simulink model "LTDung_Library2222222"  (R2016a)
settings: Solver=VariableStepAuto  SolverMode=SingleTasking  StartTime=0.0  StopTime=10.0  RelTol=1e-3
undefined symbols (not defined in the file): a, b, c, d, DiscIntNeverNeededParam, f, g, p, pe, Ts
libraries: simulink x4, powerlib_extras x2, powerlib x1
settings Model: Creator=Admin  LastModifiedBy=? ? ?
settings DebuggingCC: SFUnexpectedBacktrackingDiag=error  SFNoUnconditionalDefaultTransitionDiag=error
settings GRTTargetCC: TargetLangStandard=C99 (ISO)  GeneratePreprocessorConditionals=Use local settings
settings ConfigComp: CovMetricSettings=dwe  CovHtmlReporting=off  CovSaveCumulativeToWorkspaceVar=off  CovSaveSingleToWorkspaceVar=off  CovExternalEMLEnable=on

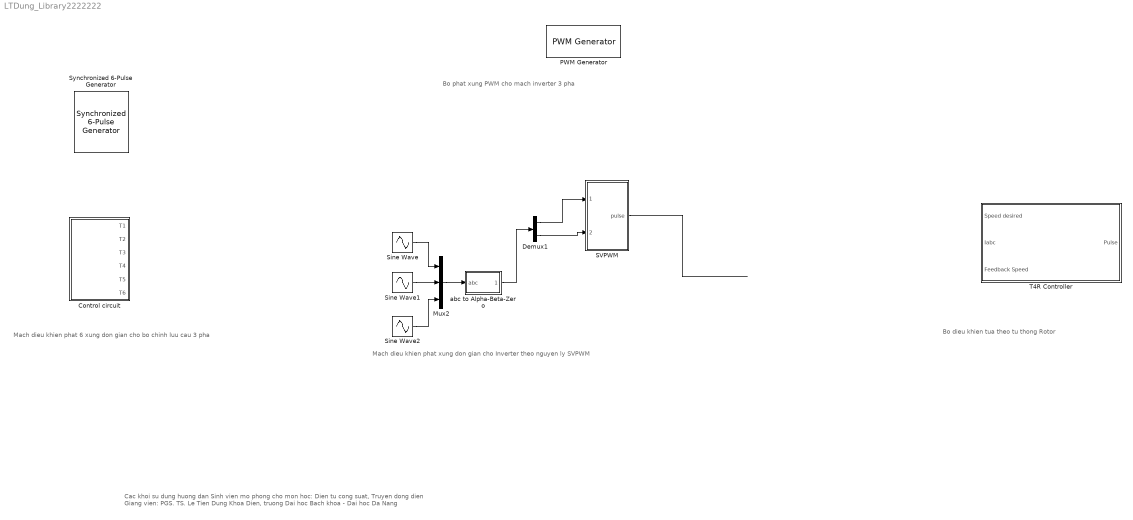
== system LTDung_Library2222222 ==
  note: Cac khoi su dung huong dan Sinh vien mo phong cho mon hoc: Dien tu cong suat, Truyen dong dien
      |
      | Giang vien: PGS. TS. Le Tien Dung
      | Khoa Dien, truong Dai hoc Bach khoa - Dai hoc Da Nang
  note: Mach dieu khien phat xung don gian cho Inverter theo nguyen ly SVPWM
  note: Mach dieu khien phat 6 xung don gian
      | cho bo chinh luu cau 3 pha
  note: Bo dieu khien tua theo tu thong Rotor
  note: Bo phat xung PWM cho mach inverter 3 pha
  Control circuit : Subsystem
  Demux1 : Demux  Outputs=2
  Mux2 : Mux  Inputs=3
  PWM Generator : powerlib_extras/Control  Blocks/PWM Generator  GeneratorMode="3-arm  bridge (6 pulses)"  Fc=5000  Internal=on  mIndex=1  Freq=50  Phase=0
  SVPWM : Subsystem
  Sine Wave : Sin  Amplitude=220*sqrt(2)  Frequency=50  SampleTime=0
  Sine Wave1 : Sin  Amplitude=220*sqrt(2)  Frequency=50  Phase=-2*pi/3  SampleTime=0
  Sine Wave2 : Sin  Amplitude=220*sqrt(2)  Frequency=50  Phase=-4*pi/3  SampleTime=0
  Synchronized 6-Pulse Generator : powerlib_extras/Control  Blocks/Synchronized 6-Pulse Generator  freq=50  pwidth=10  Double_Pulse=off
  T4R Controller : Subsystem
  abc to Alpha-Beta-Zero : Subsystem  AncestorBlock=powerlib_meascontrol/Transformations/abc to Alpha-Beta-Zero  DialogController=POWERSYS.PowerSysDialog  mask(abc to Alpha-Beta-Zero Transformation){}
      mask help: Perform a Clarke transformation from a three-phase (abc) signal to a alpha-beta-zero stationary reference frame.
      mask Help: helpview(psbhelp);
      mask Display:
      | plot([0 1], [0,1])
      | text(0.15,0.7,'abc')
      | text(0.55, 0.3,'\alpha\beta0','texmode','on')
  wires:
  Sine Wave/1 -> Mux2/1
  Demux1/1 -> SVPWM/1(Ualpha)
  abc to Alpha-Beta-Zero/1(al_be) -> Demux1/1
  Sine Wave1/1 -> Mux2/2
  Sine Wave2/1 -> Mux2/3
  Demux1/2 -> SVPWM/2(Ubeta)
  Mux2/1 -> abc to Alpha-Beta-Zero/1(abc)
  SVPWM/1(pulse) -> ?

== system LTDung_Library2222222/Control circuit ==
  Discription : Subsystem
  P1 : DiscretePulseGenerator  PulseType=Time based  Period=1/f  PulseWidth=p  PhaseDelay=((pe*a)/360)
  P2 : DiscretePulseGenerator  PulseType=Time based  Period=1/f  PulseWidth=p  PhaseDelay=((pe*b)/360)
  P3 : DiscretePulseGenerator  PulseType=Time based  Period=1/f  PulseWidth=p  PhaseDelay=((pe*c)/360)
  P4 : DiscretePulseGenerator  PulseType=Time based  Period=1/f  PulseWidth=p  PhaseDelay=((pe*d)/360)
  P5 : DiscretePulseGenerator  PulseType=Time based  Period=1/f  PulseWidth=p  PhaseDelay=((pe*e)/360)
  P6 : DiscretePulseGenerator  PulseType=Time based  Period=1/f  PulseWidth=p  PhaseDelay=((pe*g)/360)
  T1 : Outport
  T2 : Outport  Port=2
  T3 : Outport  Port=3
  T4 : Outport  Port=4
  T5 : Outport  Port=5
  T6 : Outport  Port=6
  wires:
  P4/1 -> T4/1
  P2/1 -> T2/1
  P6/1 -> T6/1
  P1/1 -> T1/1
  P5/1 -> T5/1
  P3/1 -> T3/1

== system LTDung_Library2222222/SVPWM ==
  Ualpha : Inport
  Ubeta : Inport  Port=2
  N1 : Subsystem
  Scope : Scope
  Scope1 : Scope
  Scope3 : Scope  NumInputPorts=2
  Scope6 : Scope
  Subsystem : Subsystem
  Subsystem1 : Subsystem
  T : Constant  Value=0.0001
  Udc : Constant  Value=620
  X.Y.Z : Subsystem
  produce PWM : Subsystem
  pulse : Outport
  wires:
  T/1 -> X.Y.Z/1(T), Subsystem1/3(T), Subsystem/5(T)
  Udc/1 -> X.Y.Z/4(Udc)
  N1/1(N) -> Subsystem/1(N), Subsystem1/4(N), Scope1/1
  X.Y.Z/1(X) -> Subsystem/2(X)
  X.Y.Z/2(Y) -> Subsystem/3(Y)
  X.Y.Z/3(Z) -> Subsystem/4(Z)
  Subsystem1/1(Tcm1) -> produce PWM/1(Tcm1), Scope/1
  Subsystem1/2(Tcm2) -> produce PWM/2(Tcm2)
  Subsystem1/3(Tcm3) -> produce PWM/3(Tcm3)
  Ualpha/1 -> Scope3/1, X.Y.Z/2(Ualfa), N1/1(Ualpha)
  Subsystem/1(T1) -> Subsystem1/1(T1), Scope6/1
  Subsystem/2(T2) -> Subsystem1/2(T2)
  Ubeta/1 -> X.Y.Z/3(Ubeta), N1/2(Ubeta), Scope3/2
  produce PWM/1(pulse) -> pulse/1

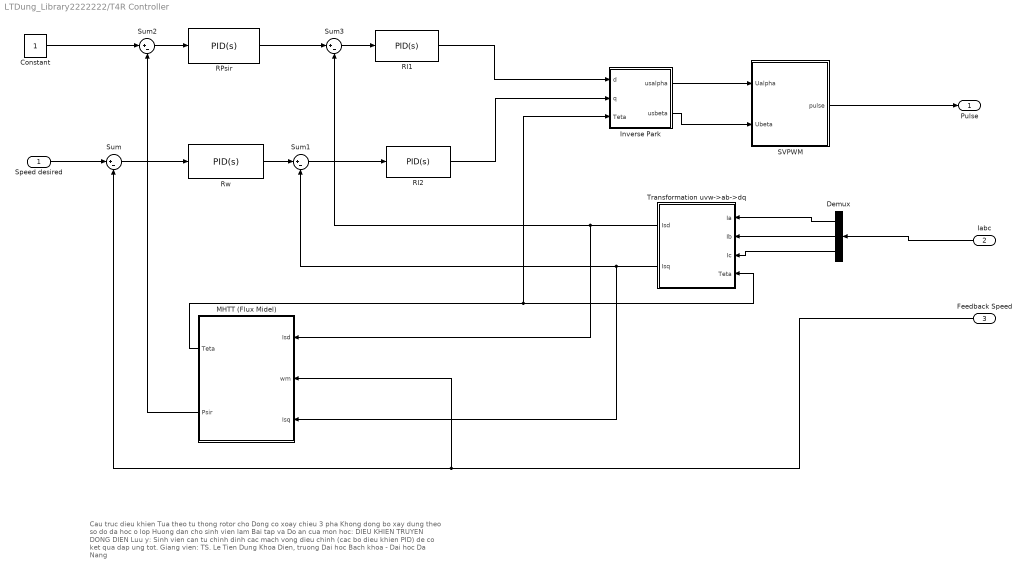
== system LTDung_Library2222222/T4R Controller ==
  note: Cau truc dieu khien Tua theo tu thong rotor cho Dong co xoay chieu 3 pha Khong dong bo xay dung theo so do da hoc o lop
      | Huong dan cho sinh vien lam Bai tap va Do an cua mon hoc: DIEU KHIEN TRUYEN DONG DIEN
      |
      | Luu y: Sinh vien can tu chinh dinh cac mach vong dieu chinh (cac bo dieu khien PID) de co ket qua dap ung tot.
      |
      | Giang vien: TS. Le Tien Dung
      | Khoa Dien, truong Dai hoc Bach khoa - Dai hoc Da Nang
  Speed desired : Inport
  Iabc : Inport  Port=2
  Feedback Speed : Inport  Port=3
  Constant : Constant
  Demux : Demux  Outputs=3
  Inverse Park : Subsystem
  MHTT (Flux Midel) : Subsystem
  RI1 : simulink/Continuous/PID Controller  Controller=PID  Form=Parallel  TimeDomain=Continuous-time  SampleTime=-1  IntegratorMethod=Forward Euler  FilterMethod=Forward Euler  ControllerParametersSource=internal  P=1  I=1  D=0  UseFilter=on  N=100  InitialConditionSource=internal  InitialConditionForIntegrator=0  InitialConditionForFilter=0  DifferentiatorICPrevScaledInput=0  ExternalReset=none  TrackingMode=off  Kt=1  LimitOutput=off  UpperSaturationLimit=inf  LowerSaturationLimit=-inf  LinearizeAsGain=on  AntiWindupMode=none  Kb=1  POutMin=[]  POutMax=[]  IOutMin=[]  IOutMax=[]  DOutMin=[]  DOutMax=[]  NOutMin=[]  NOutMax=[]  SumOutMin=[]  SumOutMax=[]  SaturationOutMin=[]  SaturationOutMax=[]  PParamMin=[]  PParamMax=[]  IParamMin=[]  IParamMax=[]  DParamMin=[]  DParamMax=[]  NParamMin=[]  NParamMax=[]  KbParamMin=[]  KbParamMax=[]  KtParamMin=[]  KtParamMax=[]  KbOutMin=[]  KbOutMax=[]  KtOutMin=[]  KtOutMax=[]  IntegratorOutMin=[]  IntegratorOutMax=[]  FilterOutMin=[]  FilterOutMax=[]  SumI1OutMin=[]  SumI1OutMax=[]  SumI2OutMin=[]  SumI2OutMax=[]  SumI3OutMin=[]  SumI3OutMax=[]  SumDOutMin=[]  SumDOutMax=[]  DifferentiatorOutMin=[]  DifferentiatorOutMax=[]  IntegratorContinuousStateAttributes=''  IntegratorStateMustResolveToSignalObject=off  IntegratorRTWStateStorageClass=Auto  FilterContinuousStateAttributes=''  FilterStateMustResolveToSignalObject=off  FilterRTWStateStorageClass=Auto
  RI2 : simulink/Continuous/PID Controller  Controller=PID  Form=Parallel  TimeDomain=Continuous-time  SampleTime=-1  IntegratorMethod=Forward Euler  FilterMethod=Forward Euler  ControllerParametersSource=internal  P=1  I=1  D=0  UseFilter=on  N=100  InitialConditionSource=internal  InitialConditionForIntegrator=0  InitialConditionForFilter=0  DifferentiatorICPrevScaledInput=0  ExternalReset=none  TrackingMode=off  Kt=1  LimitOutput=off  UpperSaturationLimit=inf  LowerSaturationLimit=-inf  LinearizeAsGain=on  AntiWindupMode=none  Kb=1  POutMin=[]  POutMax=[]  IOutMin=[]  IOutMax=[]  DOutMin=[]  DOutMax=[]  NOutMin=[]  NOutMax=[]  SumOutMin=[]  SumOutMax=[]  SaturationOutMin=[]  SaturationOutMax=[]  PParamMin=[]  PParamMax=[]  IParamMin=[]  IParamMax=[]  DParamMin=[]  DParamMax=[]  NParamMin=[]  NParamMax=[]  KbParamMin=[]  KbParamMax=[]  KtParamMin=[]  KtParamMax=[]  KbOutMin=[]  KbOutMax=[]  KtOutMin=[]  KtOutMax=[]  IntegratorOutMin=[]  IntegratorOutMax=[]  FilterOutMin=[]  FilterOutMax=[]  SumI1OutMin=[]  SumI1OutMax=[]  SumI2OutMin=[]  SumI2OutMax=[]  SumI3OutMin=[]  SumI3OutMax=[]  SumDOutMin=[]  SumDOutMax=[]  DifferentiatorOutMin=[]  DifferentiatorOutMax=[]  IntegratorContinuousStateAttributes=''  IntegratorStateMustResolveToSignalObject=off  IntegratorRTWStateStorageClass=Auto  FilterContinuousStateAttributes=''  FilterStateMustResolveToSignalObject=off  FilterRTWStateStorageClass=Auto
  RPsir : simulink/Continuous/PID Controller  Controller=PID  Form=Parallel  TimeDomain=Continuous-time  SampleTime=-1  IntegratorMethod=Forward Euler  FilterMethod=Forward Euler  ControllerParametersSource=internal  P=1  I=1  D=0  UseFilter=on  N=100  InitialConditionSource=internal  InitialConditionForIntegrator=0  InitialConditionForFilter=0  DifferentiatorICPrevScaledInput=0  ExternalReset=none  TrackingMode=off  Kt=1  LimitOutput=off  UpperSaturationLimit=inf  LowerSaturationLimit=-inf  LinearizeAsGain=on  AntiWindupMode=none  Kb=1  POutMin=[]  POutMax=[]  IOutMin=[]  IOutMax=[]  DOutMin=[]  DOutMax=[]  NOutMin=[]  NOutMax=[]  SumOutMin=[]  SumOutMax=[]  SaturationOutMin=[]  SaturationOutMax=[]  PParamMin=[]  PParamMax=[]  IParamMin=[]  IParamMax=[]  DParamMin=[]  DParamMax=[]  NParamMin=[]  NParamMax=[]  KbParamMin=[]  KbParamMax=[]  KtParamMin=[]  KtParamMax=[]  KbOutMin=[]  KbOutMax=[]  KtOutMin=[]  KtOutMax=[]  IntegratorOutMin=[]  IntegratorOutMax=[]  FilterOutMin=[]  FilterOutMax=[]  SumI1OutMin=[]  SumI1OutMax=[]  SumI2OutMin=[]  SumI2OutMax=[]  SumI3OutMin=[]  SumI3OutMax=[]  SumDOutMin=[]  SumDOutMax=[]  DifferentiatorOutMin=[]  DifferentiatorOutMax=[]  IntegratorContinuousStateAttributes=''  IntegratorStateMustResolveToSignalObject=off  IntegratorRTWStateStorageClass=Auto  FilterContinuousStateAttributes=''  FilterStateMustResolveToSignalObject=off  FilterRTWStateStorageClass=Auto
  Rw : simulink/Continuous/PID Controller  Controller=PID  Form=Parallel  TimeDomain=Continuous-time  SampleTime=-1  IntegratorMethod=Forward Euler  FilterMethod=Forward Euler  ControllerParametersSource=internal  P=1  I=1  D=0  UseFilter=on  N=100  InitialConditionSource=internal  InitialConditionForIntegrator=0  InitialConditionForFilter=0  DifferentiatorICPrevScaledInput=0  ExternalReset=none  TrackingMode=off  Kt=1  LimitOutput=off  UpperSaturationLimit=inf  LowerSaturationLimit=-inf  LinearizeAsGain=on  AntiWindupMode=none  Kb=1  POutMin=[]  POutMax=[]  IOutMin=[]  IOutMax=[]  DOutMin=[]  DOutMax=[]  NOutMin=[]  NOutMax=[]  SumOutMin=[]  SumOutMax=[]  SaturationOutMin=[]  SaturationOutMax=[]  PParamMin=[]  PParamMax=[]  IParamMin=[]  IParamMax=[]  DParamMin=[]  DParamMax=[]  NParamMin=[]  NParamMax=[]  KbParamMin=[]  KbParamMax=[]  KtParamMin=[]  KtParamMax=[]  KbOutMin=[]  KbOutMax=[]  KtOutMin=[]  KtOutMax=[]  IntegratorOutMin=[]  IntegratorOutMax=[]  FilterOutMin=[]  FilterOutMax=[]  SumI1OutMin=[]  SumI1OutMax=[]  SumI2OutMin=[]  SumI2OutMax=[]  SumI3OutMin=[]  SumI3OutMax=[]  SumDOutMin=[]  SumDOutMax=[]  DifferentiatorOutMin=[]  DifferentiatorOutMax=[]  IntegratorContinuousStateAttributes=''  IntegratorStateMustResolveToSignalObject=off  IntegratorRTWStateStorageClass=Auto  FilterContinuousStateAttributes=''  FilterStateMustResolveToSignalObject=off  FilterRTWStateStorageClass=Auto
  SVPWM : Subsystem
  Sum{,1..3} (4 alike) : Sum  Inputs=|+-
  Transformation uvw->ab->dq : Subsystem
  Pulse : Outport
  wires:
  Speed desired/1 -> Sum/1
  Sum/1 -> Rw/1
  Rw/1 -> Sum1/1
  Sum1/1 -> RI2/1
  RI2/1 -> Inverse Park/2(q)
  Constant/1 -> Sum2/1
  Sum2/1 -> RPsir/1
  RPsir/1 -> Sum3/1
  Sum3/1 -> RI1/1
  RI1/1 -> Inverse Park/1(d)
  Inverse Park/1(usalpha) -> SVPWM/1(Ualpha)
  Inverse Park/2(usbeta) -> SVPWM/2(Ubeta)
  SVPWM/1(pulse) -> Pulse/1
  Feedback Speed/1 -> MHTT (Flux Midel)/2(wm), Sum/2
  Demux/1 -> Transformation uvw->ab->dq/1(Ia)
  Demux/2 -> Transformation uvw->ab->dq/2(Ib)
  Iabc/1 -> Demux/1
  Demux/3 -> Transformation uvw->ab->dq/3(Ic)
  MHTT (Flux Midel)/2(Psir) -> Sum2/2
  MHTT (Flux Midel)/1(Teta) -> Transformation uvw->ab->dq/4(Teta), Inverse Park/3(Teta)
  Transformation uvw->ab->dq/2(Isq) -> MHTT (Flux Midel)/3(Isq), Sum1/2
  Transformation uvw->ab->dq/1(Isd) -> MHTT (Flux Midel)/1(Isd), Sum3/2

== system LTDung_Library2222222/abc to Alpha-Beta-Zero ==
  abc : Inport  PortDimensions=3
  Gain3 : Gain  Gain="[ 1   -1/2   -1/2; 0   sqrt(3)/2   -sqrt(3)/2]"  Multiplication=Matrix(K*u) (u vector)  SaturateOnIntegerOverflow=on  OutDataTypeStr=Inherit: Same as input  ParamDataTypeStr=Inherit: Same as input
  al_be : Outport
  wires:
  abc/1 -> Gain3/1
  Gain3/1 -> al_be/1

== system LTDung_Library2222222/Control circuit/Discription ==
  note: Equation
      |
      | period	= 1/fundamental frequency
      | 		= 1/50
      |
      | phase delay= (period*degree)/360
      |
      | eg	= ((0.02*60)/360)
  note: a=0
      | b=60
      | c=120
      | d=180
      | e=240
      | g=300
  powergui : powerlib/powergui  Priority=1  SimulationMode=Continuous  SampleTime=50e-6  frequency=60  Iterations=50  frequencyindice=0  Pbase=100e6  ErrMax=1e-4  UnitsV=kV  UnitsW=MW  buscounter=0  FunctionMessages=off  echomessages=off  EnableUseOfTLC=off  CurrentSourceSwitches=off  DisableSnubberDevices=off  DisableRonSwitches=off  DisableVfSwitches=off  DisplayEquations=off  SolverType=Tustin/Backward Euler (TBE)  Interpol=off  ExternalGateDelay=off  methode=off  Ts=100  x0status=blocks  SPID=on  SwTol=0  HookPort=off  RestoreLinks=warning  ResistiveCurrentMeasurement=off  Frange=[0:2:500]  Ylog=off  Xlog=on  ShowGrid=off  save=off  variable=ZData  structure=GG  ZoomFFT=off  StartTime=0.02  cycles=1  DisplayStyle=1  fundamental=25  FreqAxis=on  MaxFrequency=1000  frequencyindicesteady=1  RmsSteady=1  display=off

== system LTDung_Library2222222/SVPWM/N1 ==
  Ualpha : Inport
  Ubeta : Inport  Port=2
  Constant : Constant
  Constant1 : Constant  Value=0
  Gain : Gain  Gain=1.732
  Gain1 : Gain  Gain=-1.732
  Gain2 : Gain  Gain=2
  Gain3 : Gain  Gain=4
  Sum : Sum  Inputs=|-+
  Sum1 : Sum  Inputs=|-+
  Sum2 : Sum  Inputs=|+++
  Switch : Switch
  Switch1 : Switch
  Switch2 : Switch
  N : Outport
  wires:
  Ubeta/1 -> Switch/2, Sum/1, Sum1/1
  Constant/1 -> Switch/1, Switch2/1, Switch1/1
  Ualpha/1 -> Gain1/1, Gain/1
  Gain/1 -> Sum/2
  Sum/1 -> Switch1/2
  Sum1/1 -> Switch2/2
  Gain1/1 -> Sum1/2
  Constant1/1 -> Switch/3, Switch1/3, Switch2/3
  Switch1/1 -> Gain2/1
  Switch2/1 -> Gain3/1
  Gain2/1 -> Sum2/2
  Switch/1 -> Sum2/1
  Gain3/1 -> Sum2/3
  Sum2/1 -> N/1

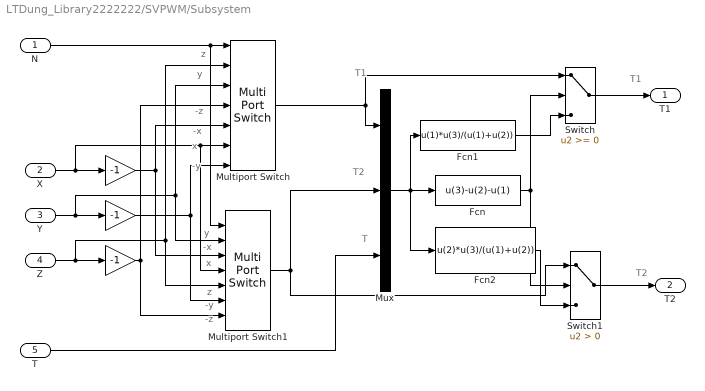
== system LTDung_Library2222222/SVPWM/Subsystem ==
  note: z
  note: y
  note: -z
  note: -x
  note: x
  note: -y
  note: y
  note: -x
  note: x
  note: z
  note: -y
  note: -z
  note: T1
  note: T2
  note: T
  note: T1
  note: T2
  N : Inport
  X : Inport  Port=2
  Y : Inport  Port=3
  Z : Inport  Port=4
  T : Inport  Port=5
  " " : Gain  Gain=-1
  "  " : Gain  Gain=-1
  "    " : Gain  Gain=-1
  Fcn : Fcn  Expr=u(3)-u(2)-u(1)
  Fcn1 : Fcn  Expr=u(1)*u(3)/(u(1)+u(2))
  Fcn2 : Fcn  Expr=u(2)*u(3)/(u(1)+u(2))
  Multiport Switch : MultiPortSwitch  Inputs=6
  Multiport Switch1 : MultiPortSwitch  Inputs=6
  Mux : Mux  Inputs=3
  Switch : Switch
  Switch1 : Switch  Criteria=u2 > Threshold
  T1 : Outport
  T2 : Outport  Port=2
  wires:
  N/1 -> Multiport Switch1/1, Multiport Switch/1
  X/1 -> Multiport Switch1/4, Multiport Switch/6, " "/1
  Y/1 -> Multiport Switch1/2, Multiport Switch/3, "  "/1
  Z/1 -> Multiport Switch1/5, Multiport Switch/2, "    "/1
  "    "/1 -> Multiport Switch1/7, Multiport Switch/4
  "  "/1 -> Multiport Switch/7, Multiport Switch1/6
  " "/1 -> Multiport Switch/5, Multiport Switch1/3
  Multiport Switch/1 -> Mux/1, Switch/1
  Multiport Switch1/1 -> Switch1/1, Mux/2
  T/1 -> Mux/3
  Mux/1 -> Fcn/1, Fcn1/1, Fcn2/1
  Fcn/1 -> Switch/2, Switch1/2
  Fcn1/1 -> Switch/3
  Fcn2/1 -> Switch1/3
  Switch/1 -> T1/1
  Switch1/1 -> T2/1

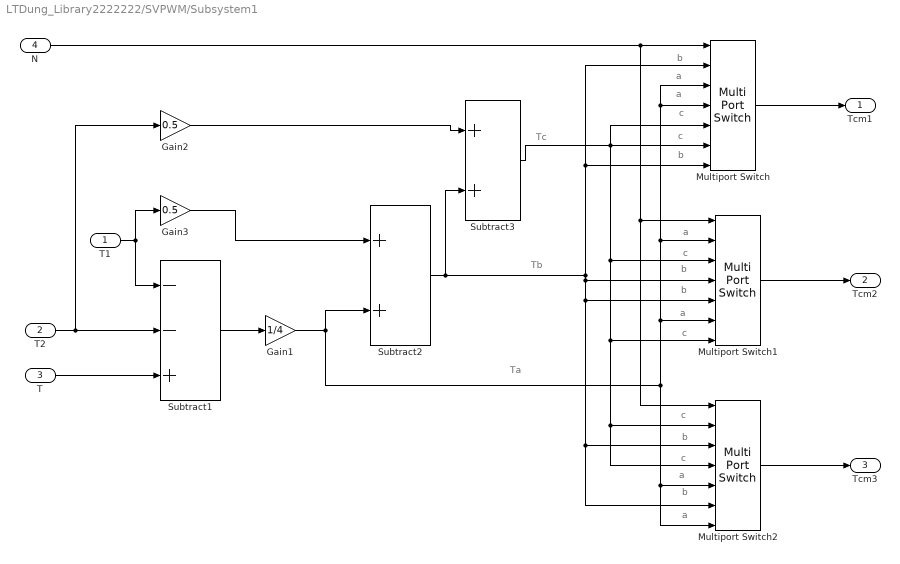
== system LTDung_Library2222222/SVPWM/Subsystem1 ==
  note: Ta
  note: Tb
  note: Tc
  note: b
  note: a
  note: a
  note: c
  note: c
  note: b
  note: a
  note: c
  note: b
  note: b
  note: a
  note: c
  note: c
  note: b
  note: c
  note: a
  note: b
  note: a
  T1 : Inport
  T2 : Inport  Port=2
  T : Inport  Port=3
  N : Inport  Port=4
  Gain1 : Gain  Gain=1/4
  Gain2 : Gain  Gain=0.5
  Gain3 : Gain  Gain=0.5
  Multiport Switch : MultiPortSwitch  Inputs=6
  Multiport Switch1 : MultiPortSwitch  Inputs=6
  Multiport Switch2 : MultiPortSwitch  Inputs=6
  Subtract1 : Sum  Inputs=--+
  Subtract2 : Sum
  Subtract3 : Sum
  Tcm1 : Outport
  Tcm2 : Outport  Port=2
  Tcm3 : Outport  Port=3
  wires:
  T2/1 -> Gain2/1, Subtract1/2
  T/1 -> Subtract1/3
  T1/1 -> Gain3/1, Subtract1/1
  Gain3/1 -> Subtract2/1
  Subtract1/1 -> Gain1/1
  Gain1/1 -> Subtract2/2, Multiport Switch/3, Multiport Switch/4, Multiport Switch1/2, Multiport Switch1/6, Multiport Switch2/5, Multiport Switch2/7
  Subtract2/1 -> Subtract3/2, Multiport Switch/2, Multiport Switch/7, Multiport Switch1/4, Multiport Switch1/5, Multiport Switch2/3, Multiport Switch2/6
  Gain2/1 -> Subtract3/1
  N/1 -> Multiport Switch/1, Multiport Switch2/1, Multiport Switch1/1
  Multiport Switch/1 -> Tcm1/1
  Multiport Switch1/1 -> Tcm2/1
  Multiport Switch2/1 -> Tcm3/1
  Subtract3/1 -> Multiport Switch/5, Multiport Switch/6, Multiport Switch1/3, Multiport Switch1/7, Multiport Switch2/2, Multiport Switch2/4

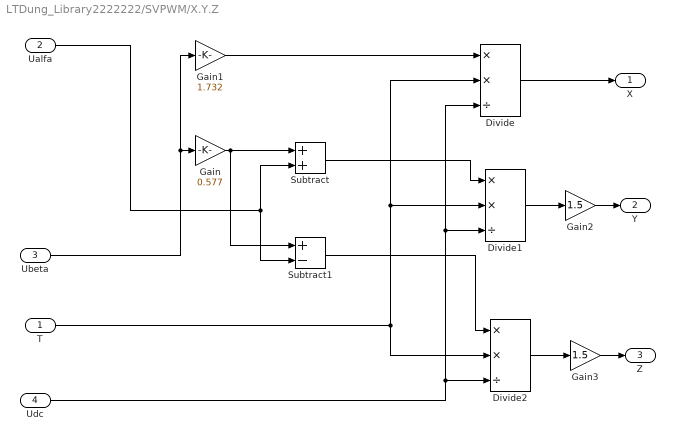
== system LTDung_Library2222222/SVPWM/X.Y.Z ==
  T : Inport
  Ualfa : Inport  Port=2
  Ubeta : Inport  Port=3
  Udc : Inport  Port=4
  Divide : Product  Inputs=**/
  Divide1 : Product  Inputs=**/
  Divide2 : Product  Inputs=**/
  Gain : Gain  Gain=0.577
  Gain1 : Gain  Gain=1.732
  Gain2 : Gain  Gain=1.5
  Gain3 : Gain  Gain=1.5
  Subtract : Sum
  Subtract1 : Sum  Inputs=+-
  X : Outport
  Y : Outport  Port=2
  Z : Outport  Port=3
  wires:
  Gain/1 -> Subtract/1, Subtract1/1
  Gain1/1 -> Divide/1
  T/1 -> Divide2/2, Divide1/2, Divide/2
  Udc/1 -> Divide2/3, Divide1/3, Divide/3
  Ualfa/1 -> Subtract1/2, Subtract/2
  Subtract/1 -> Divide1/1
  Subtract1/1 -> Divide2/1
  Divide/1 -> X/1
  Divide1/1 -> Gain2/1
  Divide2/1 -> Gain3/1
  Gain2/1 -> Y/1
  Gain3/1 -> Z/1
  Ubeta/1 -> Gain1/1, Gain/1

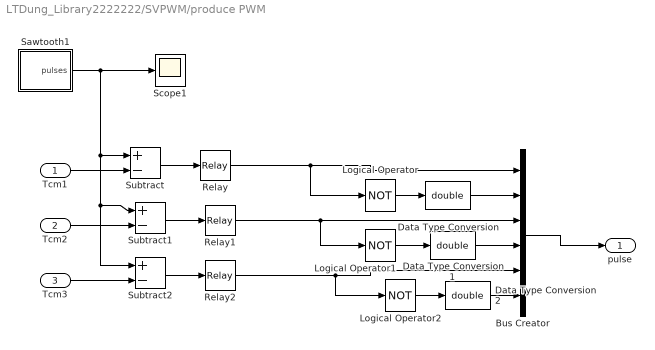
== system LTDung_Library2222222/SVPWM/produce PWM ==
  Tcm1 : Inport
  Tcm2 : Inport  Port=2
  Tcm3 : Inport  Port=3
  Bus Creator : BusCreator  Inputs=6
  Data Type Conversion : DataTypeConversion  OutDataTypeStr=double
  Data Type Conversion1 : DataTypeConversion  OutDataTypeStr=double
  Data Type Conversion2 : DataTypeConversion  OutDataTypeStr=double
  Logical Operator : Logic  Operator=NOT  AllPortsSameDT=off
  Logical Operator1 : Logic  Operator=NOT  AllPortsSameDT=off
  Logical Operator2 : Logic  Operator=NOT  AllPortsSameDT=off
  Relay : Relay
  Relay1 : Relay
  Relay2 : Relay
  Sawtooth1 : Subsystem
  Scope1 : Scope
  Subtract : Sum  Inputs=+-
  Subtract1 : Sum  Inputs=+-
  Subtract2 : Sum  Inputs=+-
  pulse : Outport
  wires:
  Subtract/1 -> Relay/1
  Subtract1/1 -> Relay1/1
  Subtract2/1 -> Relay2/1
  Sawtooth1/1(pulses) -> Subtract/1, Subtract2/1, Subtract1/1, Scope1/1
  Tcm1/1 -> Subtract/2
  Tcm2/1 -> Subtract1/2
  Tcm3/1 -> Subtract2/2
  Logical Operator1/1 -> Data Type Conversion1/1
  Logical Operator2/1 -> Data Type Conversion2/1
  Logical Operator/1 -> Data Type Conversion/1
  Relay/1 -> Bus Creator/1, Logical Operator/1
  Relay1/1 -> Bus Creator/3, Logical Operator1/1
  Relay2/1 -> Bus Creator/5, Logical Operator2/1
  Bus Creator/1 -> pulse/1
  Data Type Conversion/1 -> Bus Creator/2
  Data Type Conversion1/1 -> Bus Creator/4
  Data Type Conversion2/1 -> Bus Creator/6

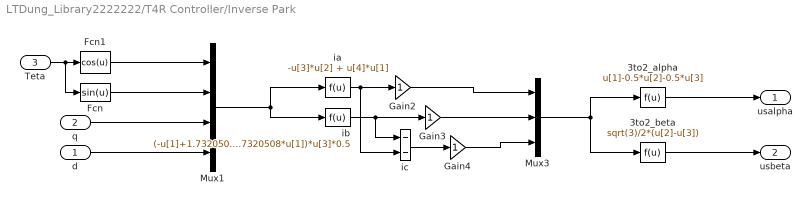
== system LTDung_Library2222222/T4R Controller/Inverse Park ==
  d : Inport
  q : Inport  Port=2
  Teta : Inport  Port=3
  3to2_alpha : Fcn  Expr=u[1]-0.5*u[2]-0.5*u[3]
  3to2_beta : Fcn  Expr=sqrt(3)/2*(u[2]-u[3])
  Fcn : Fcn  Expr=sin(u)
  Fcn1 : Fcn  Expr=cos(u)
  Gain2 : Gain  SaturateOnIntegerOverflow=on  OutDataTypeStr=Inherit: Same as input  ParamDataTypeStr=Inherit: Same as input
  Gain3 : Gain  SaturateOnIntegerOverflow=on  OutDataTypeStr=Inherit: Same as input  ParamDataTypeStr=Inherit: Same as input
  Gain4 : Gain  SaturateOnIntegerOverflow=on  OutDataTypeStr=Inherit: Same as input  ParamDataTypeStr=Inherit: Same as input
  Mux1 : Mux
  Mux3 : Mux  Inputs=3
  ia : Fcn  Expr=-u[3]*u[2] + u[4]*u[1]
  ib : Fcn  Expr=(-u[1]+1.7320508*u[2])*u[4]*0.5+(u[2]+1.7320508*u[1])*u[3]*0.5
  ic : Sum  Inputs=--  SaturateOnIntegerOverflow=on  InputSameDT=on  OutDataTypeStr=Inherit: Same as first input
  usalpha : Outport
  usbeta : Outport  Port=2
  wires:
  Fcn1/1 -> Mux1/1
  Teta/1 -> Fcn1/1, Fcn/1
  q/1 -> Mux1/3
  d/1 -> Mux1/4
  Gain3/1 -> Mux3/2
  ic/1 -> Gain4/1
  Gain4/1 -> Mux3/3
  Gain2/1 -> Mux3/1
  ia/1 -> Gain2/1, ic/2
  ib/1 -> Gain3/1, ic/1
  3to2_alpha/1 -> usalpha/1
  3to2_beta/1 -> usbeta/1
  Fcn/1 -> Mux1/2
  Mux1/1 -> ib/1, ia/1
  Mux3/1 -> 3to2_beta/1, 3to2_alpha/1

== system LTDung_Library2222222/T4R Controller/MHTT (Flux Midel) ==
  Isd : Inport
  wm : Inport  Port=2
  Isq : Inport  Port=3
  Flux Observer : Subsystem  mask(Flux Calcultation){}
      mask init:
      | NF=0.44572610323020e-6;
      | DF=[1 -0.99998715486734];
  Teta Estimator : Subsystem
  Unit Delay : UnitDelay  SampleTime=-1
  Unit Delay1 : UnitDelay  SampleTime=-1
  Teta : Outport
  Psir : Outport  Port=2
  wires:
  Unit Delay1/1 -> Teta Estimator/3(Iq)
  Teta Estimator/1(Teta) -> Teta/1
  wm/1 -> Teta Estimator/2(wm)
  Isd/1 -> Unit Delay/1
  Unit Delay/1 -> Flux Observer/1(Id)
  Flux Observer/1(Phir) -> Psir/1, Teta Estimator/1(Phird)
  Isq/1 -> Unit Delay1/1

== system LTDung_Library2222222/T4R Controller/SVPWM ==
  Ualpha : Inport
  Ubeta : Inport  Port=2
  N1 : Subsystem
  Scope : Scope
  Scope1 : Scope
  Scope3 : Scope  NumInputPorts=2
  Scope6 : Scope
  Subsystem : Subsystem
  Subsystem1 : Subsystem
  T : Constant  Value=0.0001
  Udc : Constant  Value=620
  X.Y.Z : Subsystem
  produce PWM : Subsystem
  pulse : Outport
  wires:
  T/1 -> X.Y.Z/1(T), Subsystem1/3(T), Subsystem/5(T)
  Udc/1 -> X.Y.Z/4(Udc)
  N1/1(N) -> Subsystem/1(N), Subsystem1/4(N), Scope1/1
  X.Y.Z/1(X) -> Subsystem/2(X)
  X.Y.Z/2(Y) -> Subsystem/3(Y)
  X.Y.Z/3(Z) -> Subsystem/4(Z)
  Subsystem1/1(Tcm1) -> produce PWM/1(Tcm1), Scope/1
  Subsystem1/2(Tcm2) -> produce PWM/2(Tcm2)
  Subsystem1/3(Tcm3) -> produce PWM/3(Tcm3)
  Ualpha/1 -> Scope3/1, X.Y.Z/2(Ualfa), N1/1(Ualpha)
  Subsystem/1(T1) -> Subsystem1/1(T1), Scope6/1
  Subsystem/2(T2) -> Subsystem1/2(T2)
  Ubeta/1 -> X.Y.Z/3(Ubeta), N1/2(Ubeta), Scope3/2
  produce PWM/1(pulse) -> pulse/1

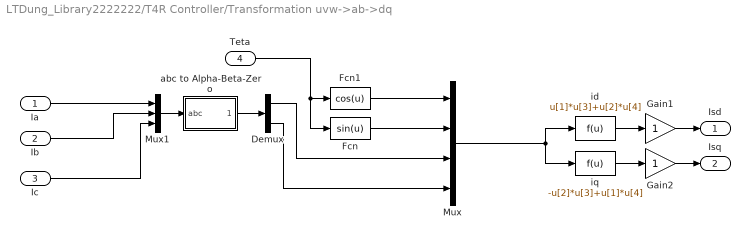
== system LTDung_Library2222222/T4R Controller/Transformation uvw->ab->dq ==
  Ia : Inport
  Ib : Inport  Port=2
  Ic : Inport  Port=3
  Teta : Inport  Port=4
  Demux : Demux  Outputs=2
  Fcn : Fcn  Expr=sin(u)
  Fcn1 : Fcn  Expr=cos(u)
  Gain1 : Gain  SaturateOnIntegerOverflow=on  OutDataTypeStr=Inherit: Same as input  ParamDataTypeStr=Inherit: Same as input
  Gain2 : Gain  SaturateOnIntegerOverflow=on  OutDataTypeStr=Inherit: Same as input  ParamDataTypeStr=Inherit: Same as input
  Mux : Mux
  Mux1 : Mux  Inputs=3
  abc to Alpha-Beta-Zero : Subsystem  AncestorBlock=powerlib_meascontrol/Transformations/abc to Alpha-Beta-Zero  DialogController=POWERSYS.PowerSysDialog  mask(abc to Alpha-Beta-Zero Transformation){}
      mask help: Perform a Clarke transformation from a three-phase (abc) signal to a alpha-beta-zero stationary reference frame.
      mask Help: helpview(psbhelp);
      mask Display:
      | plot([0 1], [0,1])
      | text(0.15,0.7,'abc')
      | text(0.55, 0.3,'\alpha\beta0','texmode','on')
  id : Fcn  Expr=u[1]*u[3]+u[2]*u[4]
  iq : Fcn  Expr=-u[2]*u[3]+u[1]*u[4]
  Isd : Outport
  Isq : Outport  Port=2
  wires:
  Ia/1 -> Mux1/1
  Ic/1 -> Mux1/3
  Mux1/1 -> abc to Alpha-Beta-Zero/1(abc)
  abc to Alpha-Beta-Zero/1(al_be) -> Demux/1
  Ib/1 -> Mux1/2
  Fcn/1 -> Mux/2
  Fcn1/1 -> Mux/1
  Mux/1 -> iq/1, id/1
  iq/1 -> Gain2/1
  id/1 -> Gain1/1
  Gain1/1 -> Isd/1
  Teta/1 -> Fcn/1, Fcn1/1
  Gain2/1 -> Isq/1
  Demux/1 -> Mux/3
  Demux/2 -> Mux/4

== system LTDung_Library2222222/SVPWM/produce PWM/Sawtooth1 ==
  Integrator : Integrator
  Pulse Generator : DiscretePulseGenerator  PulseType=Time based  Period=0.0001  PulseWidth=50
  Sum1 : Sum  Inputs=-+|  SaturateOnIntegerOverflow=on  InputSameDT=on  OutDataTypeStr=Inherit: Same as first input
  modulation index2 : Gain  Gain=2  SaturateOnIntegerOverflow=on  OutDataTypeStr=Inherit: Same as input  ParamDataTypeStr=Inherit: Same as input
  pi/1 : Constant
  pulses : Outport
  wires:
  pi/1/1 -> Sum1/1
  modulation index2/1 -> Sum1/2
  Sum1/1 -> Integrator/1
  Integrator/1 -> pulses/1
  Pulse Generator/1 -> modulation index2/1

== system LTDung_Library2222222/T4R Controller/MHTT (Flux Midel)/Flux Observer ==
  note: Phir = Lm *Id / (1 +Tr .s)
  note: Lm = 34.7 mH
  note: Lr = Ll'r +Lm = 0.8 +34.7= 35.5 mH
  note: Tr = Lr / Rr = 0.1557 s
  note: Rr = 0.228 ohms
  Id : Inport
  Discrete Tranfer Function : Subsystem  mask(First Order Low Pass Filter (Discrete)){T=0.1557, Ts=0.001}
      mask prompts: T "Time constant T (s) :"; Ts "Time step (s)"
      mask help: H(s)=1/(1+T.s)
      mask init:
      | X=[0 1 2 3 4];
      |  Y=[-2 -2 -3 -4 -4];
      |  str=sprintf('\nH=1/(1+T.s)\n T= %g s\n\n\n',T);
      | num=1;
      | den=[T 1];
      | 
      | % discrete transfer function
      | % descending powers of z
      | numd= Ts/T;
      | dend=[ 1  (Ts-T)/T];
      mask Display:
      | plot(X,Y);
      | disp(str);
  Lm : Gain  Gain=34.7e-3  SaturateOnIntegerOverflow=on  OutDataTypeStr=Inherit: Same as input  ParamDataTypeStr=Inherit: Same as input
  Phir : Outport
  wires:
  Discrete Tranfer Function/1(Out) -> Phir/1
  Id/1 -> Lm/1
  Lm/1 -> Discrete Tranfer Function/1(In)

== system LTDung_Library2222222/T4R Controller/MHTT (Flux Midel)/Teta Estimator ==
  note: Teta= Electrical angle= integ ( wr + wm)
  note: wr = Rotor frequency (rad/s) = Lm *Iq / ( Tr * Phir)
  note: Lm = 34.7 mH
  note: Rr= 0.228 ohms
  note: Lr = Ll'r +Lm = 0.8 +34.7= 35.5 mH
  note: wm= Rotor mechanical speed (rad/s)
  note: Tr = Lr / Rr = 0.1557 s
  Phird : Inport
  wm : Inport  Port=2
  Iq : Inport  Port=3
  Discrete-Time Integrator : DiscreteIntegrator  SampleTime=Ts  ICPrevOutput=DiscIntNeverNeededParam  ICPrevScaledInput=DiscIntNeverNeededParam
  Fcn : Fcn  Expr=34.7e-3*u[1]/(u[2]*0.1557+1e-3)
  Gain2 : Gain  SaturateOnIntegerOverflow=on  OutDataTypeStr=Inherit: Same as input  ParamDataTypeStr=Inherit: Same as input
  Gain3 : Gain  Gain=2  SaturateOnIntegerOverflow=on  OutDataTypeStr=Inherit: Same as input  ParamDataTypeStr=Inherit: Same as input
  Mux1 : Mux  Inputs=2
  Sum : Sum  SaturateOnIntegerOverflow=on  InputSameDT=on  OutDataTypeStr=Inherit: Same as first input
  Teta : Outport  InitialOutput=0
  wires:
  Discrete-Time Integrator/1 -> Teta/1
  Sum/1 -> Discrete-Time Integrator/1
  Gain3/1 -> Sum/2
  Gain2/1 -> Sum/1
  wm/1 -> Gain3/1
  Fcn/1 -> Gain2/1
  Phird/1 -> Mux1/2
  Iq/1 -> Mux1/1
  Mux1/1 -> Fcn/1

== system LTDung_Library2222222/T4R Controller/SVPWM/N1 ==
  Ualpha : Inport
  Ubeta : Inport  Port=2
  Constant : Constant
  Constant1 : Constant  Value=0
  Gain : Gain  Gain=1.732
  Gain1 : Gain  Gain=-1.732
  Gain2 : Gain  Gain=2
  Gain3 : Gain  Gain=4
  Sum : Sum  Inputs=|-+
  Sum1 : Sum  Inputs=|-+
  Sum2 : Sum  Inputs=|+++
  Switch : Switch
  Switch1 : Switch
  Switch2 : Switch
  N : Outport
  wires:
  Ubeta/1 -> Switch/2, Sum/1, Sum1/1
  Constant/1 -> Switch/1, Switch2/1, Switch1/1
  Ualpha/1 -> Gain1/1, Gain/1
  Gain/1 -> Sum/2
  Sum/1 -> Switch1/2
  Sum1/1 -> Switch2/2
  Gain1/1 -> Sum1/2
  Constant1/1 -> Switch/3, Switch1/3, Switch2/3
  Switch1/1 -> Gain2/1
  Switch2/1 -> Gain3/1
  Gain2/1 -> Sum2/2
  Switch/1 -> Sum2/1
  Gain3/1 -> Sum2/3
  Sum2/1 -> N/1

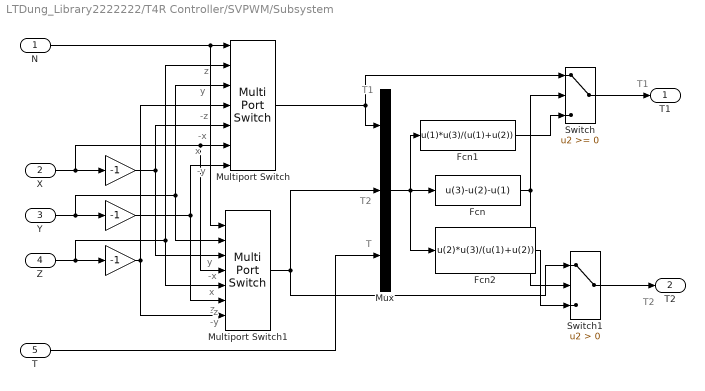
== system LTDung_Library2222222/T4R Controller/SVPWM/Subsystem ==
  note: z
  note: y
  note: -z
  note: -x
  note: x
  note: -y
  note: y
  note: -x
  note: x
  note: z
  note: -y
  note: -z
  note: T1
  note: T2
  note: T
  note: T1
  note: T2
  N : Inport
  X : Inport  Port=2
  Y : Inport  Port=3
  Z : Inport  Port=4
  T : Inport  Port=5
  " " : Gain  Gain=-1
  "  " : Gain  Gain=-1
  "    " : Gain  Gain=-1
  Fcn : Fcn  Expr=u(3)-u(2)-u(1)
  Fcn1 : Fcn  Expr=u(1)*u(3)/(u(1)+u(2))
  Fcn2 : Fcn  Expr=u(2)*u(3)/(u(1)+u(2))
  Multiport Switch : MultiPortSwitch  Inputs=6  DiagnosticForDefault=None
  Multiport Switch1 : MultiPortSwitch  Inputs=6  DiagnosticForDefault=None
  Mux : Mux  Inputs=3
  Switch : Switch
  Switch1 : Switch  Criteria=u2 > Threshold
  T1 : Outport
  T2 : Outport  Port=2
  wires:
  N/1 -> Multiport Switch1/1, Multiport Switch/1
  X/1 -> Multiport Switch1/4, Multiport Switch/6, " "/1
  Y/1 -> Multiport Switch1/2, Multiport Switch/3, "  "/1
  Z/1 -> Multiport Switch1/5, Multiport Switch/2, "    "/1
  "    "/1 -> Multiport Switch1/7, Multiport Switch/4
  "  "/1 -> Multiport Switch/7, Multiport Switch1/6
  " "/1 -> Multiport Switch/5, Multiport Switch1/3
  Multiport Switch/1 -> Mux/1, Switch/1
  Multiport Switch1/1 -> Switch1/1, Mux/2
  T/1 -> Mux/3
  Mux/1 -> Fcn/1, Fcn1/1, Fcn2/1
  Fcn/1 -> Switch/2, Switch1/2
  Fcn1/1 -> Switch/3
  Fcn2/1 -> Switch1/3
  Switch/1 -> T1/1
  Switch1/1 -> T2/1

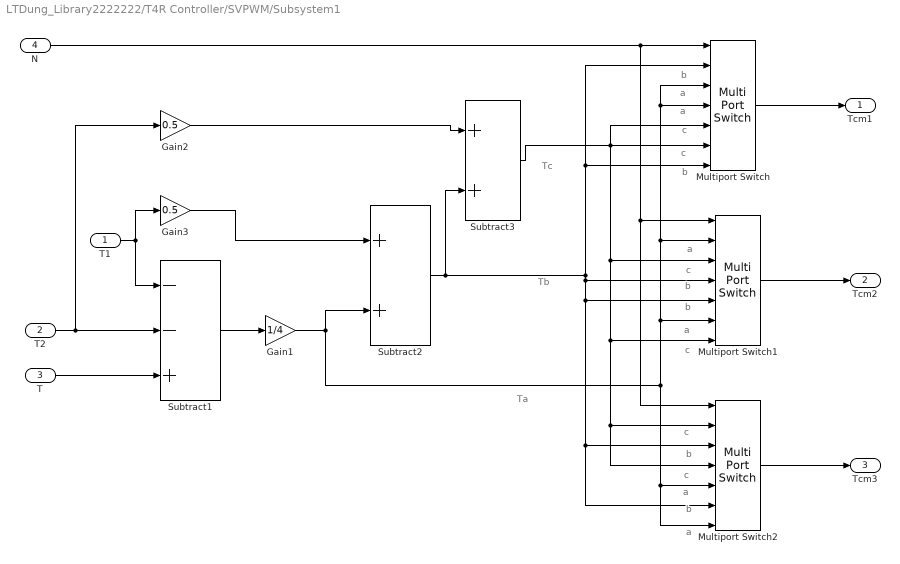
== system LTDung_Library2222222/T4R Controller/SVPWM/Subsystem1 ==
  note: Ta
  note: Tb
  note: Tc
  note: b
  note: a
  note: a
  note: c
  note: c
  note: b
  note: a
  note: c
  note: b
  note: b
  note: a
  note: c
  note: c
  note: b
  note: c
  note: a
  note: b
  note: a
  T1 : Inport
  T2 : Inport  Port=2
  T : Inport  Port=3
  N : Inport  Port=4
  Gain1 : Gain  Gain=1/4
  Gain2 : Gain  Gain=0.5
  Gain3 : Gain  Gain=0.5
  Multiport Switch : MultiPortSwitch  Inputs=6  DiagnosticForDefault=None
  Multiport Switch1 : MultiPortSwitch  Inputs=6  DiagnosticForDefault=None
  Multiport Switch2 : MultiPortSwitch  Inputs=6  DiagnosticForDefault=None
  Subtract1 : Sum  Inputs=--+
  Subtract2 : Sum
  Subtract3 : Sum
  Tcm1 : Outport
  Tcm2 : Outport  Port=2
  Tcm3 : Outport  Port=3
  wires:
  T2/1 -> Gain2/1, Subtract1/2
  T/1 -> Subtract1/3
  T1/1 -> Gain3/1, Subtract1/1
  Gain3/1 -> Subtract2/1
  Subtract1/1 -> Gain1/1
  Gain1/1 -> Subtract2/2, Multiport Switch/3, Multiport Switch/4, Multiport Switch1/2, Multiport Switch1/6, Multiport Switch2/5, Multiport Switch2/7
  Subtract2/1 -> Subtract3/2, Multiport Switch/2, Multiport Switch/7, Multiport Switch1/4, Multiport Switch1/5, Multiport Switch2/3, Multiport Switch2/6
  Gain2/1 -> Subtract3/1
  N/1 -> Multiport Switch/1, Multiport Switch2/1, Multiport Switch1/1
  Multiport Switch/1 -> Tcm1/1
  Multiport Switch1/1 -> Tcm2/1
  Multiport Switch2/1 -> Tcm3/1
  Subtract3/1 -> Multiport Switch/5, Multiport Switch/6, Multiport Switch1/3, Multiport Switch1/7, Multiport Switch2/2, Multiport Switch2/4

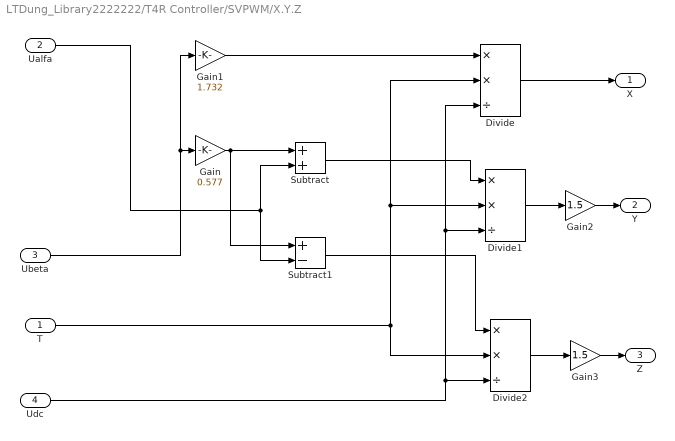
== system LTDung_Library2222222/T4R Controller/SVPWM/X.Y.Z ==
  T : Inport
  Ualfa : Inport  Port=2
  Ubeta : Inport  Port=3
  Udc : Inport  Port=4
  Divide : Product  Inputs=**/
  Divide1 : Product  Inputs=**/
  Divide2 : Product  Inputs=**/
  Gain : Gain  Gain=0.577
  Gain1 : Gain  Gain=1.732
  Gain2 : Gain  Gain=1.5
  Gain3 : Gain  Gain=1.5
  Subtract : Sum
  Subtract1 : Sum  Inputs=+-
  X : Outport
  Y : Outport  Port=2
  Z : Outport  Port=3
  wires:
  Gain/1 -> Subtract/1, Subtract1/1
  Gain1/1 -> Divide/1
  T/1 -> Divide2/2, Divide1/2, Divide/2
  Udc/1 -> Divide2/3, Divide1/3, Divide/3
  Ualfa/1 -> Subtract1/2, Subtract/2
  Subtract/1 -> Divide1/1
  Subtract1/1 -> Divide2/1
  Divide/1 -> X/1
  Divide1/1 -> Gain2/1
  Divide2/1 -> Gain3/1
  Gain2/1 -> Y/1
  Gain3/1 -> Z/1
  Ubeta/1 -> Gain1/1, Gain/1

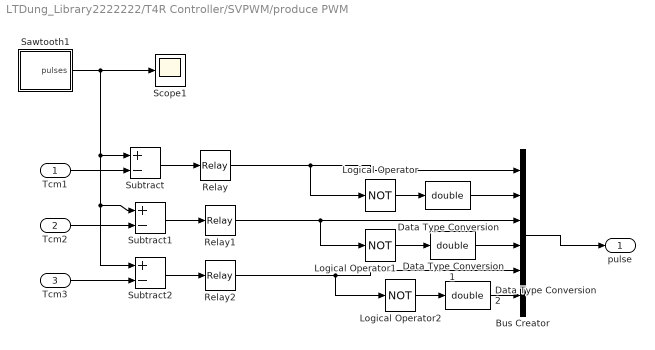
== system LTDung_Library2222222/T4R Controller/SVPWM/produce PWM ==
  Tcm1 : Inport
  Tcm2 : Inport  Port=2
  Tcm3 : Inport  Port=3
  Bus Creator : BusCreator  Inputs=6
  Data Type Conversion : DataTypeConversion  OutDataTypeStr=double
  Data Type Conversion1 : DataTypeConversion  OutDataTypeStr=double
  Data Type Conversion2 : DataTypeConversion  OutDataTypeStr=double
  Logical Operator : Logic  Operator=NOT  AllPortsSameDT=off
  Logical Operator1 : Logic  Operator=NOT  AllPortsSameDT=off
  Logical Operator2 : Logic  Operator=NOT  AllPortsSameDT=off
  Relay : Relay
  Relay1 : Relay
  Relay2 : Relay
  Sawtooth1 : Subsystem
  Scope1 : Scope
  Subtract : Sum  Inputs=+-
  Subtract1 : Sum  Inputs=+-
  Subtract2 : Sum  Inputs=+-
  pulse : Outport
  wires:
  Subtract/1 -> Relay/1
  Subtract1/1 -> Relay1/1
  Subtract2/1 -> Relay2/1
  Sawtooth1/1(pulses) -> Subtract/1, Subtract2/1, Subtract1/1, Scope1/1
  Tcm1/1 -> Subtract/2
  Tcm2/1 -> Subtract1/2
  Tcm3/1 -> Subtract2/2
  Logical Operator1/1 -> Data Type Conversion1/1
  Logical Operator2/1 -> Data Type Conversion2/1
  Logical Operator/1 -> Data Type Conversion/1
  Relay/1 -> Bus Creator/1, Logical Operator/1
  Relay1/1 -> Bus Creator/3, Logical Operator1/1
  Relay2/1 -> Bus Creator/5, Logical Operator2/1
  Bus Creator/1 -> pulse/1
  Data Type Conversion/1 -> Bus Creator/2
  Data Type Conversion1/1 -> Bus Creator/4
  Data Type Conversion2/1 -> Bus Creator/6

== system LTDung_Library2222222/T4R Controller/Transformation uvw->ab->dq/abc to Alpha-Beta-Zero ==
  abc : Inport  PortDimensions=3
  Gain3 : Gain  Gain="[ 1   -1/2   -1/2; 0   sqrt(3)/2   -sqrt(3)/2]"  Multiplication=Matrix(K*u) (u vector)  SaturateOnIntegerOverflow=on  OutDataTypeStr=Inherit: Same as input  ParamDataTypeStr=Inherit: Same as input
  al_be : Outport
  wires:
  abc/1 -> Gain3/1
  Gain3/1 -> al_be/1

== system LTDung_Library2222222/T4R Controller/MHTT (Flux Midel)/Flux Observer/Discrete Tranfer Function ==
  In : Inport
  Discrete Transfer Fcn : DiscreteTransferFcn  Numerator=numd  Denominator=dend  SampleTime=Ts
  Out : Outport  InitialOutput=0
  wires:
  Discrete Transfer Fcn/1 -> Out/1
  In/1 -> Discrete Transfer Fcn/1

== system LTDung_Library2222222/T4R Controller/SVPWM/produce PWM/Sawtooth1 ==
  Integrator : Integrator
  Pulse Generator : DiscretePulseGenerator  PulseType=Time based  Period=0.0001  PulseWidth=50
  Sum1 : Sum  Inputs=-+|  SaturateOnIntegerOverflow=on  InputSameDT=on  OutDataTypeStr=Inherit: Same as first input
  modulation index2 : Gain  Gain=2  SaturateOnIntegerOverflow=on  OutDataTypeStr=Inherit: Same as input  ParamDataTypeStr=Inherit: Same as input
  pi/1 : Constant
  pulses : Outport
  wires:
  pi/1/1 -> Sum1/1
  modulation index2/1 -> Sum1/2
  Sum1/1 -> Integrator/1
  Integrator/1 -> pulses/1
  Pulse Generator/1 -> modulation index2/1
